simulink model "untitled"  (R2021b)
settings: Solver=VariableStepAuto  StartTime=0.0  StopTime=10.0  RelTol=1e-3
values from neighbouring files (symbols this model uses):
  ad = exp(-Ts*pd_param.a)    [measureFrequencyResponse.m]    (also in measureFrequencyResponse_pd.m)
  Kd = Kp*(Td-Ta)    [designPD_lead_compensator.m]    (also in designPID_lead_compensator.m = K*(Ti-Ta)*(Td-Ta); measureFrequencyResponse.m = pd_param.Kd; measureFrequencyResponse_pd.m = pd_param.Kd)
  Ki = K    [designPID_lead_compensator.m]    (also in measureFrequencyResponse.m = pd_param.Ki; measureFrequencyResponse_pd.m = pd_param.Ki)
  Kp = abs(j*w_c*Ta + 1)/( abs(j*w_c*Td + 1) * mag_G_jwc)    [designLeadCompensator.m]    (also in designPD_lead_compensator.m = lc_param.Kp; designPID_lead_compensator.m = K*(Ti+Td-Ta); measureFrequencyResponse.m = pd_param.Kp; measureFrequencyResponse_pd.m = pd_param.Kp)
  pd_param = struct()    [designPD_lead_compensator.m]    (also in init.m = designPD_lead_compensator(lc_param); pd_parameters.mat = )
  T_sample = Ts    (= 0.001)    [measureFrequencyResponse.m]    (also in measureFrequencyResponse_pd.m)
undefined symbols (not defined in the file or in its folder): DiscIntNeverNeededParam
libraries: simulink x1
settings Model: Creator=ssapkota  LastModifiedBy=ssapkota

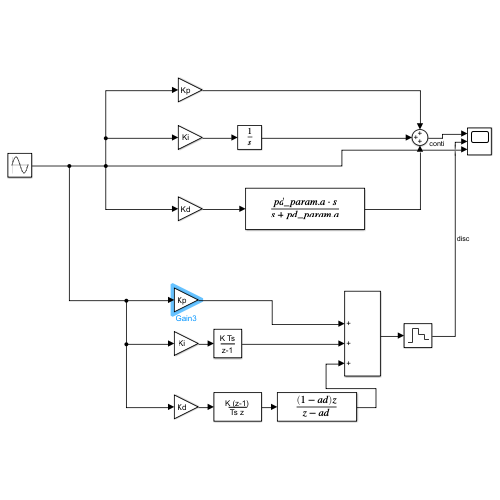
[thumbnail: Simulink's stored preview of the top-level diagram]
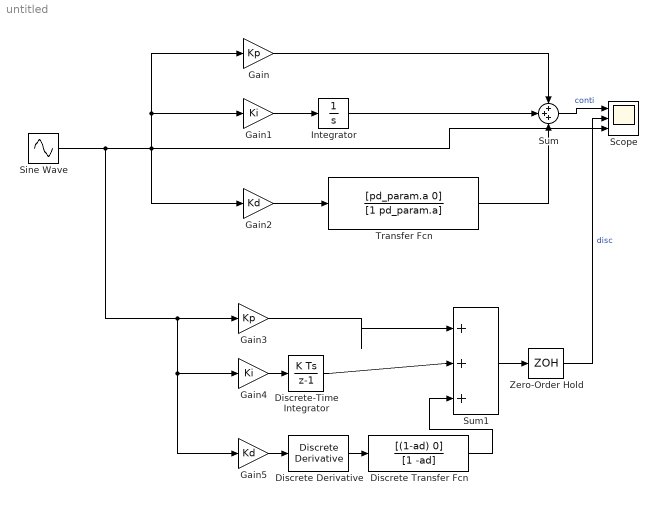
== system untitled ==
  Discrete Transfer Fcn : DiscreteTransferFcn  Numerator=[(1-ad) 0]  Denominator=[1 -ad]
  Discrete Derivative : simulink/Discrete/Discrete Derivative  gainval=1.0  ICPrevScaledInput=0.0  OutMin=[]  OutMax=[]  OutDataType=fixdt(1, 16)  OutScaling=2^-10  DoSatur=off
  Discrete-Time Integrator : DiscreteIntegrator  SampleTime=-1  ICPrevOutput=DiscIntNeverNeededParam  ICPrevScaledInput=DiscIntNeverNeededParam
  Gain : Gain  Gain=Kp
  Gain1 : Gain  Gain=Ki
  Gain2 : Gain  Gain=Kd
  Gain3 : Gain  Gain=Kp
  Gain4 : Gain  Gain=Ki
  Gain5 : Gain  Gain=Kd
  Integrator : Integrator
  Scope : Scope  NumInputPorts=3
  Sine Wave : Sin  Frequency=50  SampleTime=0
  Sum : Sum  Inputs=+++
  Sum1 : Sum  Inputs=|+++
  Transfer Fcn : TransferFcn  Numerator=[pd_param.a 0]  Denominator=[1 pd_param.a]
  Zero-Order Hold : ZeroOrderHold  SampleTime=T_sample
  wires:
  Gain1/1 -> Integrator/1
  Gain2/1 -> Transfer Fcn/1
  Transfer Fcn/1 -> Sum/3
  Integrator/1 -> Sum/2
  Gain/1 -> Sum/1
  Sum/1 -> Scope/1  "conti"
  Gain3/1 -> Sum1/1
  Discrete-Time Integrator/1 -> Sum1/2
  Gain5/1 -> Discrete Derivative/1
  Sum1/1 -> Zero-Order Hold/1
  Sine Wave/1 -> Scope/3, Gain2/1, Gain1/1, Gain/1, Gain5/1, Gain4/1, Gain3/1
  Discrete Transfer Fcn/1 -> Sum1/3
  Gain4/1 -> Discrete-Time Integrator/1
  Discrete Derivative/1 -> Discrete Transfer Fcn/1
  Zero-Order Hold/1 -> Scope/2  "disc"
